simulink model "VELO"  (R2019b)
settings: Solver=FixedStepAuto  StartTime=0.0  StopTime=t(end)  FixedStep=0.01  RelTol=1e-3
undefined symbols (not defined in the file or in its folder): dfilt, fdesignblkfcn, gcbh
libraries: eeGeneralControl x27, dspstat3 x20, dspfdesign x12, sharedTrackingLibrary x3, dsparch4 x2, dspxfrm3 x1, cstblocks x1
(part 2 of 2)

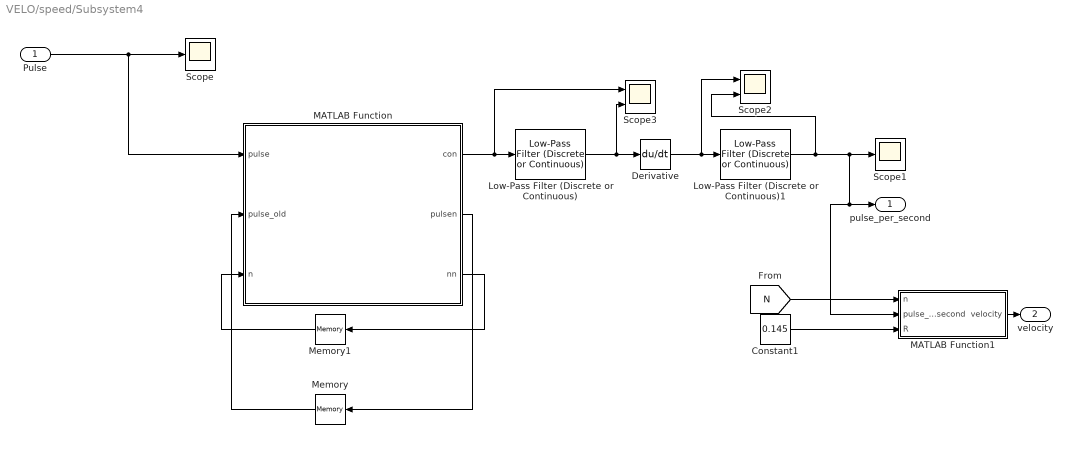
== system VELO/speed/Subsystem4 ==
  Pulse : Inport
  Constant1 : Constant  Value=0.145
  Derivative : Derivative
  Low-Pass Filter (Discrete or Continuous) : eeGeneralControl/Low-Pass Filter (Discrete or Continuous)  K=1  T=0.4  B=inf  A=-inf  Ts=-1
      settings: SourceProductName=Simscape Electrical
  Low-Pass Filter (Discrete or Continuous)1 : eeGeneralControl/Low-Pass Filter (Discrete or Continuous)  K=1  T=0.2  B=inf  A=-inf  Ts=-1
      settings: SourceProductName=Simscape Electrical
  MATLAB Function : MATLAB Function  TreatAsAtomicUnit=on
  MATLAB Function1 : MATLAB Function  TreatAsAtomicUnit=on
  Memory : Memory
  Memory1 : Memory
  Scope : Scope
  Scope1 : Scope
  Scope2 : Scope  NumInputPorts=2
  Scope3 : Scope  NumInputPorts=2
  pulse_per_second : Outport
  velocity : Outport  Port=2
  wires:
  Low-Pass Filter (Discrete or Continuous)/1 -> Derivative/1, Scope3/2
  Derivative/1 -> Low-Pass Filter (Discrete or Continuous)1/1, Scope2/1
  Memory/1 -> MATLAB Function/2(pulse_old)
  Pulse/1 -> MATLAB Function/1(pulse), Scope/1
  MATLAB Function/2(pulsen) -> Memory/1
  MATLAB Function/3(nn) -> Memory1/1
  Memory1/1 -> MATLAB Function/3(n)
  MATLAB Function/1(con) -> Scope3/1, Low-Pass Filter (Discrete or Continuous)/1
  Low-Pass Filter (Discrete or Continuous)1/1 -> pulse_per_second/1, MATLAB Function1/2(pulse_per_second), Scope1/1, Scope2/2
  [N] -> MATLAB Function1/1(n)
  Constant1/1 -> MATLAB Function1/3(R)
  MATLAB Function1/1(velocity) -> velocity/1

== system VELO/speed/Subsystem5 ==
  Moving Average{,1..3} (4 alike) : dspstat3/Moving Average  Method=Sliding window  ForgettingFactorPort=off  SpecifyWindowLength=on  WindowLength=50  ForgettingFactor=0.9  SimulateUsing=Code generation
  Mux : Mux
  Scope10 : Scope
  To Workspace : ToWorkspace  VariableName=V_Wp  SaveFormat=Timeseries  SampleTime=-1
  wires:
  [V_w4] -> Moving Average/1
  Mux/1 -> To Workspace/1, Scope10/1
  [V_w1] -> Moving Average3/1
  [V_w2] -> Moving Average2/1
  [V_w3] -> Moving Average1/1
  Moving Average/1 -> Mux/4  "v_w4"
  Moving Average1/1 -> Mux/3  "v_w3"
  Moving Average2/1 -> Mux/2  "v_w2"
  Moving Average3/1 -> Mux/1  "v_w1"

== matlab function VELO/speed/Subsystem1/MATLAB Function ==
  data: pulse input; con output; pulse_old input; n input; pulsen output; nn output
function [con ,pulsen,nn] = fcn(pulse,pulse_old,n)

if pulse<pulse_old
    
    nn=n+1;
con=nn*255+pulse;

else 
 
con=n*255+pulse;
nn=n;
end
pulsen=pulse;
end

== matlab function VELO/speed/Subsystem1/MATLAB Function1 ==
  data: n input; velocity output; pulse_per_second input; R input
function velocity = fcn(n,pulse_per_second,R)

velocity =(pulse_per_second*3.6/(2*pi*n))*R;
end

== matlab function VELO/speed/Subsystem2/MATLAB Function ==
  data: pulse input; con output; pulse_old input; n input; pulsen output; nn output
function [con ,pulsen,nn] = fcn(pulse,pulse_old,n)

if pulse<pulse_old
    
    nn=n+1;
con=nn*255+pulse;

else 
 
con=n*255+pulse;
nn=n;
end
pulsen=pulse;
end

== matlab function VELO/speed/Subsystem2/MATLAB Function1 ==
  data: n input; velocity output; pulse_per_second input; R input
function velocity = fcn(n,pulse_per_second,R)

velocity =(pulse_per_second*3.6/(2*pi*n))*R;
end

== matlab function VELO/speed/Subsystem4/MATLAB Function ==
  data: pulse input; con output; pulse_old input; n input; pulsen output; nn output
function [con ,pulsen,nn] = fcn(pulse,pulse_old,n)

if pulse<pulse_old
    
    nn=n+1;
con=nn*255+pulse;

else 
 
con=n*255+pulse;
nn=n;
end
pulsen=pulse;
end

== matlab function VELO/speed/Subsystem4/MATLAB Function1 ==
  data: n input; velocity output; pulse_per_second input; R input
function velocity = fcn(n,pulse_per_second,R)

velocity =(pulse_per_second*3.6/(2*pi*n))*R;
end

== matlab function VELO/speed/Subsystem3/MATLAB Function ==
  data: pulse input; con output; pulse_old input; n input; pulsen output; nn output
function [con ,pulsen,nn] = fcn(pulse,pulse_old,n)

if pulse<pulse_old
    
    nn=n+1;
con=nn*255+pulse;

else 
 
con=n*255+pulse;
nn=n;
end
pulsen=pulse;
end

== matlab function VELO/speed/Subsystem3/MATLAB Function1 ==
  data: n input; velocity output; pulse_per_second input; R input
function velocity = fcn(n,pulse_per_second,R)

velocity =(pulse_per_second*3.6/(2*pi*n))*R;
end

== matlab function VELO/speed/MATLAB Function ==
  data: a input; D output; b input; c input; d input
function D = fcn(a,b,c,d)

D=(a*c)/(b*d);

end

== matlab function VELO/Raw data filer /Subsystem1/MATLAB Function ==
  data: z1 input; x_hat output; z2 input; z3 input
function x_hat=fusion(z1,z2,z3)
% Kalman Filter sensor fusion example based on
%  
% http://www.slideshare.net/antoniomorancardenas/data-fusion-with-kalman-filtering
%
% % See http://home.wlu.edu/~levys/kalman_tutorial for background

% Copyright (C) 2014 Simon D. Levy
%
% This code is free software: you can redistribute it and/or modify
% it under the terms of the GNU Lesser General Public License as
% published by the Free Software Foundation, either version 3 of the
% License, or (at your option) any later version.
%
% This code is distributed in the hope that it will be useful,
% but WITHOUT ANY WARRANTY without even the implied warranty of
% MERCHANTABILITY or FITNESS FOR A PARTICULAR PURPOSE. See the
% GNU General Public License for more details.
%
% You should have received a copy of the GNU Lesser General Public License
% along with this code. If not, see <http:#www.gnu.org/licenses/>.

% Parameters ============================================================

% Biases
% BIAS1 = +1;
% BIAS2 = -1;

% Measurement noise covariances
R1 = 0.64;
R2 = 0.64;
R3 = 0.64;
% Process noise covariance
Q = .005;

% State transition model
A = 1;

% Observation model
C1 = 1;
C2 = 1;
C3=1;
% Duration
% N = 1000;

% Run ====================================================================

% Generate the signal x as a sine wave
% x = 20 + sin(5*linspace(0,1,N)*pi);

% Add some process noise with covariance Q
% w = sqrt(Q) * randn(size(x));
% x = x + w;

% Compute noisy sensor values
% z1 = BIAS1 + x + sqrt(R1) * randn(size(x));
% z2 = BIAS2 + x + sqrt(R2) * randn(size(x));

% Run a single-sensor example and plot it
% xhat = kalman(z1, A, C1, R1, Q);
% 
% % Plot sensed and estimated values
% clf
% plotsigs(1, z1, xhat, 'Sensor 1')
% title('One sensor: signal cleanup')
% 
% % Plot estimate and actual values
% plotsigsrms('One sensor', 2, x, xhat)

% Run the Kalman filter on fused sensors
x_hat = kalman([z1; z2; z3], A, [C1; C2 ;C3], [R1 0 0; 0 R2 0;0 0 R3], [Q;Q;Q]);
end

% Plot fusion example


% Helper functions ======================================================

== matlab function VELO/Raw data filer /Subsystem2/MATLAB Function ==
  data: z1 input; x_hat output; z2 input; z3 input
function x_hat=fusion(z1,z2,z3)
% Kalman Filter sensor fusion example based on
%  
% http://www.slideshare.net/antoniomorancardenas/data-fusion-with-kalman-filtering
%
% % See http://home.wlu.edu/~levys/kalman_tutorial for background

% Copyright (C) 2014 Simon D. Levy
%
% This code is free software: you can redistribute it and/or modify
% it under the terms of the GNU Lesser General Public License as
% published by the Free Software Foundation, either version 3 of the
% License, or (at your option) any later version.
%
% This code is distributed in the hope that it will be useful,
% but WITHOUT ANY WARRANTY without even the implied warranty of
% MERCHANTABILITY or FITNESS FOR A PARTICULAR PURPOSE. See the
% GNU General Public License for more details.
%
% You should have received a copy of the GNU Lesser General Public License
% along with this code. If not, see <http:#www.gnu.org/licenses/>.

% Parameters ============================================================

% Biases
% BIAS1 = +1;
% BIAS2 = -1;

% Measurement noise covariances
R1 = 0.64;
R2 = 0.64;
R3 = 0.64;
% Process noise covariance
Q = .005;

% State transition model
A = 1;

% Observation model
C1 = 1;
C2 = 1;
C3=1;
% Duration
% N = 1000;

% Run ====================================================================

% Generate the signal x as a sine wave
% x = 20 + sin(5*linspace(0,1,N)*pi);

% Add some process noise with covariance Q
% w = sqrt(Q) * randn(size(x));
% x = x + w;

% Compute noisy sensor values
% z1 = BIAS1 + x + sqrt(R1) * randn(size(x));
% z2 = BIAS2 + x + sqrt(R2) * randn(size(x));

% Run a single-sensor example and plot it
% xhat = kalman(z1, A, C1, R1, Q);
% 
% % Plot sensed and estimated values
% clf
% plotsigs(1, z1, xhat, 'Sensor 1')
% title('One sensor: signal cleanup')
% 
% % Plot estimate and actual values
% plotsigsrms('One sensor', 2, x, xhat)

% Run the Kalman filter on fused sensors
x_hat = kalman([z1; z2; z3], A, [C1; C2 ;C3], [R1 0 0; 0 R2 0;0 0 R3], [Q;Q;Q]);
end

% Plot fusion example


% Helper functions ======================================================

== matlab function VELO/Raw data filer /Subsystem3/MATLAB Function ==
  data: z1 input; x_hat output; z2 input; z3 input
function x_hat=fusion(z1,z2,z3)
% Kalman Filter sensor fusion example based on
%  
% http://www.slideshare.net/antoniomorancardenas/data-fusion-with-kalman-filtering
%
% % See http://home.wlu.edu/~levys/kalman_tutorial for background

% Copyright (C) 2014 Simon D. Levy
%
% This code is free software: you can redistribute it and/or modify
% it under the terms of the GNU Lesser General Public License as
% published by the Free Software Foundation, either version 3 of the
% License, or (at your option) any later version.
%
% This code is distributed in the hope that it will be useful,
% but WITHOUT ANY WARRANTY without even the implied warranty of
% MERCHANTABILITY or FITNESS FOR A PARTICULAR PURPOSE. See the
% GNU General Public License for more details.
%
% You should have received a copy of the GNU Lesser General Public License
% along with this code. If not, see <http:#www.gnu.org/licenses/>.

% Parameters ============================================================

% Biases
% BIAS1 = +1;
% BIAS2 = -1;

% Measurement noise covariances
R1 = 0.64;
R2 = 0.64;
R3 = 0.64;
% Process noise covariance
Q = .005;

% State transition model
A = 1;

% Observation model
C1 = 1;
C2 = 1;
C3=1;
% Duration
% N = 1000;

% Run ====================================================================

% Generate the signal x as a sine wave
% x = 20 + sin(5*linspace(0,1,N)*pi);

% Add some process noise with covariance Q
% w = sqrt(Q) * randn(size(x));
% x = x + w;

% Compute noisy sensor values
% z1 = BIAS1 + x + sqrt(R1) * randn(size(x));
% z2 = BIAS2 + x + sqrt(R2) * randn(size(x));

% Run a single-sensor example and plot it
% xhat = kalman(z1, A, C1, R1, Q);
% 
% % Plot sensed and estimated values
% clf
% plotsigs(1, z1, xhat, 'Sensor 1')
% title('One sensor: signal cleanup')
% 
% % Plot estimate and actual values
% plotsigsrms('One sensor', 2, x, xhat)

% Run the Kalman filter on fused sensors
x_hat = kalman([z1; z2; z3], A, [C1; C2 ;C3], [R1 0 0; 0 R2 0;0 0 R3], [Q;Q;Q]);
end

% Plot fusion example


% Helper functions ======================================================

== matlab function VELO/Raw data filer /Subsystem4/MATLAB Function ==
  data: z1 input; x_hat output; z2 input; z3 input
function x_hat=fusion(z1,z2,z3)
% Kalman Filter sensor fusion example based on
%  
% http://www.slideshare.net/antoniomorancardenas/data-fusion-with-kalman-filtering
%
% % See http://home.wlu.edu/~levys/kalman_tutorial for background

% Copyright (C) 2014 Simon D. Levy
%
% This code is free software: you can redistribute it and/or modify
% it under the terms of the GNU Lesser General Public License as
% published by the Free Software Foundation, either version 3 of the
% License, or (at your option) any later version.
%
% This code is distributed in the hope that it will be useful,
% but WITHOUT ANY WARRANTY without even the implied warranty of
% MERCHANTABILITY or FITNESS FOR A PARTICULAR PURPOSE. See the
% GNU General Public License for more details.
%
% You should have received a copy of the GNU Lesser General Public License
% along with this code. If not, see <http:#www.gnu.org/licenses/>.

% Parameters ============================================================

% Biases
% BIAS1 = +1;
% BIAS2 = -1;

% Measurement noise covariances
R1 = 0.64;
R2 = 0.64;
R3 = 0.64;
% Process noise covariance
Q = .005;

% State transition model
A = 1;

% Observation model
C1 = 1;
C2 = 1;
C3=1;
% Duration
% N = 1000;

% Run ====================================================================

% Generate the signal x as a sine wave
% x = 20 + sin(5*linspace(0,1,N)*pi);

% Add some process noise with covariance Q
% w = sqrt(Q) * randn(size(x));
% x = x + w;

% Compute noisy sensor values
% z1 = BIAS1 + x + sqrt(R1) * randn(size(x));
% z2 = BIAS2 + x + sqrt(R2) * randn(size(x));

% Run a single-sensor example and plot it
% xhat = kalman(z1, A, C1, R1, Q);
% 
% % Plot sensed and estimated values
% clf
% plotsigs(1, z1, xhat, 'Sensor 1')
% title('One sensor: signal cleanup')
% 
% % Plot estimate and actual values
% plotsigsrms('One sensor', 2, x, xhat)

% Run the Kalman filter on fused sensors
x_hat = kalman([z1; z2; z3], A, [C1; C2 ;C3], [R1 0 0; 0 R2 0;0 0 R3], [Q;Q;Q]);
end

% Plot fusion example


% Helper functions ======================================================

== matlab function VELO/Raw data filer /Subsystem5/MATLAB Function ==
  data: z1 input; x_hat output; z2 input; z3 input
function x_hat=fusion(z1,z2,z3)
% Kalman Filter sensor fusion example based on
%  
% http://www.slideshare.net/antoniomorancardenas/data-fusion-with-kalman-filtering
%
% % See http://home.wlu.edu/~levys/kalman_tutorial for background

% Copyright (C) 2014 Simon D. Levy
%
% This code is free software: you can redistribute it and/or modify
% it under the terms of the GNU Lesser General Public License as
% published by the Free Software Foundation, either version 3 of the
% License, or (at your option) any later version.
%
% This code is distributed in the hope that it will be useful,
% but WITHOUT ANY WARRANTY without even the implied warranty of
% MERCHANTABILITY or FITNESS FOR A PARTICULAR PURPOSE. See the
% GNU General Public License for more details.
%
% You should have received a copy of the GNU Lesser General Public License
% along with this code. If not, see <http:#www.gnu.org/licenses/>.

% Parameters ============================================================

% Biases
% BIAS1 = +1;
% BIAS2 = -1;

% Measurement noise covariances
R1 = 0.64;
R2 = 0.64;
R3 = 0.64;
% Process noise covariance
Q = .005;

% State transition model
A = 1;

% Observation model
C1 = 1;
C2 = 1;
C3=1;
% Duration
% N = 1000;

% Run ====================================================================

% Generate the signal x as a sine wave
% x = 20 + sin(5*linspace(0,1,N)*pi);

% Add some process noise with covariance Q
% w = sqrt(Q) * randn(size(x));
% x = x + w;

% Compute noisy sensor values
% z1 = BIAS1 + x + sqrt(R1) * randn(size(x));
% z2 = BIAS2 + x + sqrt(R2) * randn(size(x));

% Run a single-sensor example and plot it
% xhat = kalman(z1, A, C1, R1, Q);
% 
% % Plot sensed and estimated values
% clf
% plotsigs(1, z1, xhat, 'Sensor 1')
% title('One sensor: signal cleanup')
% 
% % Plot estimate and actual values
% plotsigsrms('One sensor', 2, x, xhat)

% Run the Kalman filter on fused sensors
x_hat = kalman([z1; z2; z3], A, [C1; C2 ;C3], [R1 0 0; 0 R2 0;0 0 R3], [Q;Q;Q]);
end

% Plot fusion example


% Helper functions ======================================================

== matlab function VELO/Raw data filer /Subsystem6/MATLAB Function ==
  data: z1 input; x_hat output; z2 input; z3 input
function x_hat=fusion(z1,z2,z3)
% Kalman Filter sensor fusion example based on
%  
% http://www.slideshare.net/antoniomorancardenas/data-fusion-with-kalman-filtering
%
% % See http://home.wlu.edu/~levys/kalman_tutorial for background

% Copyright (C) 2014 Simon D. Levy
%
% This code is free software: you can redistribute it and/or modify
% it under the terms of the GNU Lesser General Public License as
% published by the Free Software Foundation, either version 3 of the
% License, or (at your option) any later version.
%
% This code is distributed in the hope that it will be useful,
% but WITHOUT ANY WARRANTY without even the implied warranty of
% MERCHANTABILITY or FITNESS FOR A PARTICULAR PURPOSE. See the
% GNU General Public License for more details.
%
% You should have received a copy of the GNU Lesser General Public License
% along with this code. If not, see <http:#www.gnu.org/licenses/>.

% Parameters ============================================================

% Biases
% BIAS1 = +1;
% BIAS2 = -1;

% Measurement noise covariances
R1 = 0.64;
R2 = 0.64;
R3 = 0.64;
% Process noise covariance
Q = .005;

% State transition model
A = 1;

% Observation model
C1 = 1;
C2 = 1;
C3=1;
% Duration
% N = 1000;

% Run ====================================================================

% Generate the signal x as a sine wave
% x = 20 + sin(5*linspace(0,1,N)*pi);

% Add some process noise with covariance Q
% w = sqrt(Q) * randn(size(x));
% x = x + w;

% Compute noisy sensor values
% z1 = BIAS1 + x + sqrt(R1) * randn(size(x));
% z2 = BIAS2 + x + sqrt(R2) * randn(size(x));

% Run a single-sensor example and plot it
% xhat = kalman(z1, A, C1, R1, Q);
% 
% % Plot sensed and estimated values
% clf
% plotsigs(1, z1, xhat, 'Sensor 1')
% title('One sensor: signal cleanup')
% 
% % Plot estimate and actual values
% plotsigsrms('One sensor', 2, x, xhat)

% Run the Kalman filter on fused sensors
x_hat = kalman([z1; z2; z3], A, [C1; C2 ;C3], [R1 0 0; 0 R2 0;0 0 R3], [Q;Q;Q]);
end

% Plot fusion example


% Helper functions ======================================================

== matlab function VELO/Subsystem3/MATLAB Function ==
  data: z1 input; x_hat output; z2 input; z3 input
function x_hat=fusion(z1,z2,z3)
% Kalman Filter sensor fusion example based on
%  
% http://www.slideshare.net/antoniomorancardenas/data-fusion-with-kalman-filtering
%
% % See http://home.wlu.edu/~levys/kalman_tutorial for background

% Copyright (C) 2014 Simon D. Levy
%
% This code is free software: you can redistribute it and/or modify
% it under the terms of the GNU Lesser General Public License as
% published by the Free Software Foundation, either version 3 of the
% License, or (at your option) any later version.
%
% This code is distributed in the hope that it will be useful,
% but WITHOUT ANY WARRANTY without even the implied warranty of
% MERCHANTABILITY or FITNESS FOR A PARTICULAR PURPOSE. See the
% GNU General Public License for more details.
%
% You should have received a copy of the GNU Lesser General Public License
% along with this code. If not, see <http:#www.gnu.org/licenses/>.

% Parameters ============================================================

% Biases
% BIAS1 = +1;
% BIAS2 = -1;

% Measurement noise covariances
R1 = 0.1;
R2 = 0.7;
R3 = 0.1;
% Process noise covariance
Q = .005;

% State transition model
A = 1;

% Observation model
C1 = 1;
C2 = 1;
C3=1;
% Duration
% N = 1000;

% Run ====================================================================

% Generate the signal x as a sine wave
% x = 20 + sin(5*linspace(0,1,N)*pi);

% Add some process noise with covariance Q
% w = sqrt(Q) * randn(size(x));
% x = x + w;

% Compute noisy sensor values
% z1 = BIAS1 + x + sqrt(R1) * randn(size(x));
% z2 = BIAS2 + x + sqrt(R2) * randn(size(x));

% Run a single-sensor example and plot it
% xhat = kalman(z1, A, C1, R1, Q);
% 
% % Plot sensed and estimated values
% clf
% plotsigs(1, z1, xhat, 'Sensor 1')
% title('One sensor: signal cleanup')
% 
% % Plot estimate and actual values
% plotsigsrms('One sensor', 2, x, xhat)

% Run the Kalman filter on fused sensors
x_hat = kalman([z1; z2; z3], A, [C1; C2 ;C3], [R1 0 0; 0 R2 0;0 0 R3], [Q;Q;Q]);
end

% Plot fusion example


% Helper functions ======================================================

== matlab function VELO/speed/MATLAB Function1 ==
  data: z1 input; x_hat output; z2 input; z3 input
function x_hat=fusion(z1,z2,z3)
% Kalman Filter sensor fusion example based on
%  
% http://www.slideshare.net/antoniomorancardenas/data-fusion-with-kalman-filtering
%
% % See http://home.wlu.edu/~levys/kalman_tutorial for background

% Copyright (C) 2014 Simon D. Levy
%
% This code is free software: you can redistribute it and/or modify
% it under the terms of the GNU Lesser General Public License as
% published by the Free Software Foundation, either version 3 of the
% License, or (at your option) any later version.
%
% This code is distributed in the hope that it will be useful,
% but WITHOUT ANY WARRANTY without even the implied warranty of
% MERCHANTABILITY or FITNESS FOR A PARTICULAR PURPOSE. See the
% GNU General Public License for more details.
%
% You should have received a copy of the GNU Lesser General Public License
% along with this code. If not, see <http:#www.gnu.org/licenses/>.

% Parameters ============================================================

% Biases
% BIAS1 = +1;
% BIAS2 = -1;

% Measurement noise covariances
R1 = 0.64;
R2 = 0.64;
R3 = 0.64;
% Process noise covariance
Q = .005;

% State transition model
A = 1;

% Observation model
C1 = 1;
C2 = 1;
C3=1;
% Duration
% N = 1000;

% Run ====================================================================

% Generate the signal x as a sine wave
% x = 20 + sin(5*linspace(0,1,N)*pi);

% Add some process noise with covariance Q
% w = sqrt(Q) * randn(size(x));
% x = x + w;

% Compute noisy sensor values
% z1 = BIAS1 + x + sqrt(R1) * randn(size(x));
% z2 = BIAS2 + x + sqrt(R2) * randn(size(x));

% Run a single-sensor example and plot it
% xhat = kalman(z1, A, C1, R1, Q);
% 
% % Plot sensed and estimated values
% clf
% plotsigs(1, z1, xhat, 'Sensor 1')
% title('One sensor: signal cleanup')
% 
% % Plot estimate and actual values
% plotsigsrms('One sensor', 2, x, xhat)

% Run the Kalman filter on fused sensors
x_hat = kalman([z1; z2; z3], A, [C1; C2 ;C3], [R1 0 0; 0 R2 0;0 0 R3], [Q;Q;Q]);
end

% Plot fusion example


% Helper functions ======================================================

== matlab function VELO/pitch roll yaw dispacement/MATLAB Function1 ==
  data: v_w input; s output; v_v input
function s = fcn(v_w,v_v)

s =100* (-v_w+v_v)/(v_v);
end

== matlab function VELO/Subsystem1/MATLAB Function ==
  data: ax input; a output; ay input; az input
function a = fcn(ax,ay,az)
a=sqrt(ax^2+ay^2+az^2);
end

== matlab function VELO/MATLAB Function ==
  data: ax input; teta0 output; az input; ay input; phi0 output
function [teta0,phi0] = fcn(ax,az,ay)

teta0=atan(ax/az);
phi0=atan(ay/az);

end

== matlab function VELO/Raw data filer /MATLAB Function1 ==
  data: ax input; az_pp output; ay input; az input; ax_pp output; ay_pp output; teta0 input; phi0 input; psi0 input; a_abs input
function [az_pp,ax_pp,ay_pp] = fcn(ax,ay,az,teta0,phi0,psi0,a_abs)
gain=1/a_abs;

az_p=az*cos(teta0)+ax*sin(teta0);
ax_p=ax*cos(teta0)-az*sin(teta0);

az_pp=gain*(az_p*cos(phi0)+ay*sin(phi0));
ay_p=ay*cos(phi0)-az_p*sin(phi0);
ax_pp=gain*(ax_p*cos(psi0)+ay_p*sin(psi0));
ay_pp=gain*(ay_p*cos(psi0)-ax_p*sin(psi0));
end

== matlab function VELO/Raw data filer /MATLAB Function2 ==
  data: ax input; az_pp output; ay input; az input; ax_pp output; ay_pp output; teta0 input; phi0 input; psi0 input; a_abs input
function [az_pp,ax_pp,ay_pp] = fcn(ax,ay,az,teta0,phi0,psi0,a_abs)
gain=1/a_abs;

az_p=az*cos(teta0)+ax*sin(teta0);
ax_p=ax*cos(teta0)-az*sin(teta0);

az_pp=gain*(az_p*cos(phi0)+ay*sin(phi0));
ay_p=ay*cos(phi0)-az_p*sin(phi0);
ax_pp=gain*(ax_p*cos(psi0)+ay_p*sin(psi0));
ay_pp=gain*(ay_p*cos(psi0)-ax_p*sin(psi0));
end

== matlab function VELO/MATLAB Function2 ==
  data: accz input; grade output
function grade = fcn(accz)

grade=(400/pi)*acos(accz/1);
end

== matlab function VELO/MATLAB Function1 ==
  data: graden input; ay input; ax input; az input; grade0 input; grade output; flag output
function [grade,flag] = fcn(graden,ay,ax,az,grade0)
if abs(ay)<=0.051&& abs(ax)<=0.051 && abs(az)<=1
    grade=graden;
    flag=1;
else
    grade=grade0;
flag=0;
end

end

== matlab function VELO/Raw data filer /MATLAB Function ==
  data: az input; theta output
function theta = fcn(az)
ARG=(1.0210418-abs(az))/1.0210418;
if ARG>=1
    ARG=0.01;
end
if ARG<=-1
    ARG=-0.01;
end
ARG
theta=asin(ARG)*4000/pi;
end

== matlab function VELO/Longitudinal Force Est./MATLAB Function ==
  data: Ax input; Fx output; Vx input; m input
function Fx = fcn(Ax, Vx, m)

g = 9.81;
Da = 0.5*0.29*1.22*2.01; % Aerodynamics overall coefficient
fR = 0.01; % Rolling resistance coefficient
Fr = fR*m*g;

if Ax >= 0
    
    Fx = m*abs(Ax) + abs(Fr) + abs(Da*Vx^2);
    
else
    
    Fx = (m*abs(Ax) - abs(Fr) - abs(Da*Vx^2)) / 2; % When braking, both front and rear axles are engaged

end

== matlab function VELO/Longitudinal Force Est./MATLAB Function1 ==
  data: Ax input; Fx output; Vx input; m input
function Fx = fcn(Ax, Vx, m)

g = 9.81;

Da = 0.5*0.29*1.22*2.01; % Aerodynamics overall coefficient
fR = 0.01; % Rolling resistance coefficient
Fr = fR*m*g;

if Ax >= 0
    
    Fx = m*abs(Ax) + abs(Fr) + abs(Da*Vx^2);
    
else
    
    Fx = (m*abs(Ax) - abs(Fr) - abs(Da*Vx^2)) / 2; % When braking, both front and rear axles are engaged
        
end

== matlab function VELO/Normal Force Est./MATLAB Function ==
  data: Ax input; Fzf output; Vx input; m input; Fzr output
function [Fzf, Fzr] = fcn(Ax, Vx, m)

g = 9.81;
Lf = 0.95;
Lr = 1.53;
h = 0.36;
ha = 0.62;

Da = 0.5*0.29*1.225*2.01; % Aerodynamics overall coefficient
L = Lf + Lr;
    
Fzf = (m*g*Lr - m*Ax*h - ha*Da*Vx^2)/L;
    
Fzr = (m*g*Lf + m*Ax*h + ha*Da*Vx^2)/L;
        
end

== matlab function VELO/Normal Force Est./MATLAB Function1 ==
  data: Ax input; Fzf output; Vx input; m input; Fzr output
function [Fzf, Fzr] = fcn(Ax, Vx, m)

g = 9.81;
Lf = 0.95;
Lr = 1.53;
h = 0.36;
ha = 0.62;

Da = 0.5*0.29*1.225*2.01; % Aerodynamics overall coefficient

% Da = 0.4; % Aerodynamics overall coefficient
L = Lf + Lr;
    
Fzf = (m*g*Lr - m*Ax*h - ha*Da*Vx^2)/L;
    
Fzr = (m*g*Lf + m*Ax*h + ha*Da*Vx^2)/L;
        
end
